simulink model "carsim_vxvy_force"  (R2021a)
settings: Solver=ode45  StartTime=0.0  StopTime=25  RelTol=1e-4
model workspace (MAT data in the model file):
  Freq = 1
values from neighbouring files (symbols this model uses):
  actuator_param = [mu_steer wn_steer csi_steer tau_steer mu_force wn_force csi_force tau_force]    [singletrack_beta_force_fialawos_ideal.m]    (also in singletrack_beta_force_fialawos_real.m; singletrack_beta_force_fialaws_ideal.m; singletrack_beta_force_fialaws_real.m; singletrack_beta_force_linear_ideal.m)
  car_param = [a b m mu Cf Cr Iz]    [singletrack_beta_force_fialawos_ideal.m]    (also in singletrack_beta_force_fialawos_real.m; singletrack_beta_force_fialaws_ideal.m; singletrack_beta_force_fialaws_real.m; singletrack_beta_force_linear_ideal.m)
  Fxr_ref = timeseries(ode_res.Fxr_ref,ode_res.t)    [singletrack_beta_force_fialawos_ideal.m]    (also in singletrack_beta_force_fialawos_real.m; singletrack_beta_force_fialaws_ideal.m; singletrack_beta_force_fialaws_real.m; singletrack_beta_force_linear_ideal.m)
  initial_state = [v0 beta0 r0 psi0 x0 y0]    [singletrack_beta_force_fialawos_ideal.m]    (also in singletrack_beta_force_fialawos_real.m; singletrack_beta_force_fialaws_ideal.m; singletrack_beta_force_fialaws_real.m; singletrack_beta_force_linear_ideal.m)
  steer_ref = timeseries(ode_res.steer_ref,ode_res.t)    [singletrack_beta_force_fialawos_ideal.m]    (also in singletrack_beta_force_fialawos_real.m; singletrack_beta_force_fialaws_ideal.m; singletrack_beta_force_fialaws_real.m; singletrack_beta_force_linear_ideal.m)
  Ts = ode_res.t(2)-ode_res.t(1)    [singletrack_beta_force_fialawos_ideal.m]    (also in singletrack_beta_force_fialawos_real.m; singletrack_beta_force_fialaws_ideal.m; singletrack_beta_force_fialaws_real.m; singletrack_beta_force_linear_ideal.m)
  tyre_model = 2    [singletrack_beta_force_fialawos_ideal.m]    (also in singletrack_beta_force_fialawos_real.m; singletrack_beta_force_fialaws_ideal.m = 1; singletrack_beta_force_fialaws_real.m = 1; singletrack_beta_force_linear_ideal.m = 0)
settings Model: Creator=bascetta  LastModifiedBy=bascetta
settings SolverCC: AlgebraicLoopSolver=TrustRegion  DecoupledContinuousIntegration=on
settings DataIOCC: SaveOutput=off  SignalLogging=off  DSMLogging=off  SaveTime=off  ReturnWorkspaceOutputs=off
settings DebuggingCC: ReadBeforeWriteMsg=DisableAll  WriteAfterWriteMsg=DisableAll  WriteAfterReadMsg=DisableAll  MultiTaskDSMMsg=none  SFMachineParentedDataDiag=warning  ArithmeticOperatorsInVariantConditions=warning
settings ModelReferenceCC: UpdateModelReferenceTargets=IfOutOfDate
settings SFSimCC: SFSimEcho=off  SimUseLocalCustomCode=off  CustomCodeUndefinedFunction=UseInterfaceOnly
settings RTWCC: RTWUseLocalCustomCode=off

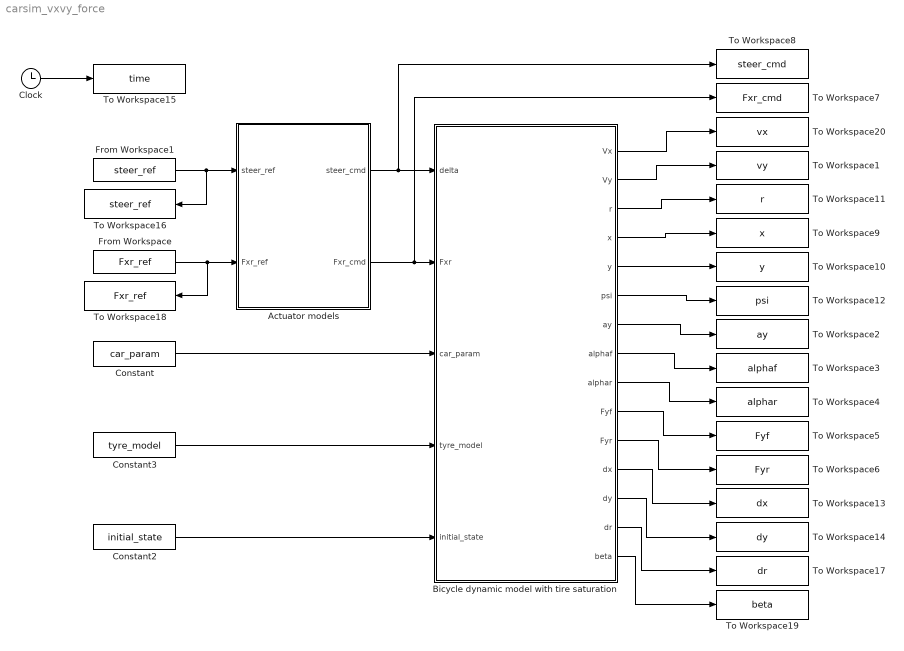
== system carsim_vxvy_force ==
  Actuator models : Subsystem  mask{mu_steer=actuator_param(1), wn_steer=actuator_param(2), csi_steer=actuator_param(3), tau_steer=actuator_param(4), steer_initial=steer_ref.Data(1), mu_force=actuator_param(5), wn_force=actuator_param(6), csi_force=actuator_param(7), tau_force=actuator_param(8), force_initial=Fxr_ref.Data(1)}
      mask prompts: mu_steer "Gain"; wn_steer "Natural frequency"; csi_steer "Damping"; tau_steer "Delay"; steer_initial "Initial value"; mu_force "Gain"; wn_force "Natural frequency"; csi_force "Damping"; tau_force "Delay"; force_initial "Initial value"
      mask DialogControl Container3 Prompt: Steer actuator parameters
      mask DialogControl Container4 Prompt: Speed actuator parameters
  Bicycle dynamic model with tire saturation : Subsystem
  Clock : Clock
  Constant : Constant  Value=car_param
  Constant2 : Constant  Value=initial_state
  Constant3 : Constant  Value=tyre_model
  From Workspace : FromWorkspace  VariableName=Fxr_ref
  From Workspace1 : FromWorkspace  VariableName=steer_ref
  To Workspace1 : ToWorkspace  VariableName=vy  SampleTime=Ts
      settings: Save2DSignal=2-D array (concatenate along first dimension)
  To Workspace10 : ToWorkspace  VariableName=y  SampleTime=Ts
      settings: Save2DSignal=2-D array (concatenate along first dimension)
  To Workspace11 : ToWorkspace  VariableName=r  SampleTime=Ts
      settings: Save2DSignal=2-D array (concatenate along first dimension)
  To Workspace12 : ToWorkspace  VariableName=psi  SampleTime=Ts
      settings: Save2DSignal=2-D array (concatenate along first dimension)
  To Workspace13 : ToWorkspace  VariableName=dx  SampleTime=Ts
      settings: Save2DSignal=2-D array (concatenate along first dimension)
  To Workspace14 : ToWorkspace  VariableName=dy  SampleTime=Ts
      settings: Save2DSignal=2-D array (concatenate along first dimension)
  To Workspace15 : ToWorkspace  VariableName=time  SampleTime=Ts
      settings: Save2DSignal=2-D array (concatenate along first dimension)
  To Workspace16 : ToWorkspace  VariableName=steer_ref  SampleTime=Ts
      settings: Save2DSignal=2-D array (concatenate along first dimension)
  To Workspace17 : ToWorkspace  VariableName=dr  SampleTime=Ts
      settings: Save2DSignal=2-D array (concatenate along first dimension)
  To Workspace18 : ToWorkspace  VariableName=Fxr_ref  SampleTime=Ts
      settings: Save2DSignal=2-D array (concatenate along first dimension)
  To Workspace19 : ToWorkspace  VariableName=beta  SampleTime=Ts
      settings: Save2DSignal=2-D array (concatenate along first dimension)
  To Workspace2 : ToWorkspace  VariableName=ay  SampleTime=Ts
      settings: Save2DSignal=2-D array (concatenate along first dimension)
  To Workspace20 : ToWorkspace  VariableName=vx  SampleTime=Ts
      settings: Save2DSignal=2-D array (concatenate along first dimension)
  To Workspace3 : ToWorkspace  VariableName=alphaf  SampleTime=Ts
      settings: Save2DSignal=2-D array (concatenate along first dimension)
  To Workspace4 : ToWorkspace  VariableName=alphar  SampleTime=Ts
      settings: Save2DSignal=2-D array (concatenate along first dimension)
  To Workspace5 : ToWorkspace  VariableName=Fyf  SampleTime=Ts
      settings: Save2DSignal=2-D array (concatenate along first dimension)
  To Workspace6 : ToWorkspace  VariableName=Fyr  SampleTime=Ts
      settings: Save2DSignal=2-D array (concatenate along first dimension)
  To Workspace7 : ToWorkspace  VariableName=Fxr_cmd  SampleTime=Ts
      settings: Save2DSignal=2-D array (concatenate along first dimension)
  To Workspace8 : ToWorkspace  VariableName=steer_cmd  SampleTime=Ts
      settings: Save2DSignal=2-D array (concatenate along first dimension)
  To Workspace9 : ToWorkspace  VariableName=x  SampleTime=Ts
      settings: Save2DSignal=2-D array (concatenate along first dimension)
  wires:
  Bicycle dynamic model with tire saturation/2(Vy) -> To Workspace1/1
  Bicycle dynamic model with tire saturation/3(r) -> To Workspace11/1
  Bicycle dynamic model with tire saturation/7(ay) -> To Workspace2/1
  Bicycle dynamic model with tire saturation/8(alphaf) -> To Workspace3/1
  Bicycle dynamic model with tire saturation/9(alphar) -> To Workspace4/1
  Bicycle dynamic model with tire saturation/10(Fyf) -> To Workspace5/1
  Bicycle dynamic model with tire saturation/11(Fyr) -> To Workspace6/1
  Constant/1 -> Bicycle dynamic model with tire saturation/3(car_param)
  Constant2/1 -> Bicycle dynamic model with tire saturation/5("initial_state ")
  Constant3/1 -> Bicycle dynamic model with tire saturation/4(tyre_model)
  Actuator models/1(steer_cmd) -> To Workspace8/1, Bicycle dynamic model with tire saturation/1(delta)
  Actuator models/2(Fxr_cmd) -> To Workspace7/1, Bicycle dynamic model with tire saturation/2(Fxr)
  From Workspace/1 -> To Workspace18/1, Actuator models/2(Fxr_ref)
  From Workspace1/1 -> To Workspace16/1, Actuator models/1(steer_ref)
  Bicycle dynamic model with tire saturation/4(x) -> To Workspace9/1
  Bicycle dynamic model with tire saturation/5(y) -> To Workspace10/1
  Bicycle dynamic model with tire saturation/6(psi) -> To Workspace12/1
  Bicycle dynamic model with tire saturation/12(dx) -> To Workspace13/1
  Bicycle dynamic model with tire saturation/13(dy) -> To Workspace14/1
  Clock/1 -> To Workspace15/1
  Bicycle dynamic model with tire saturation/14(dr) -> To Workspace17/1
  Bicycle dynamic model with tire saturation/15(beta) -> To Workspace19/1
  Bicycle dynamic model with tire saturation/1(Vx) -> To Workspace20/1

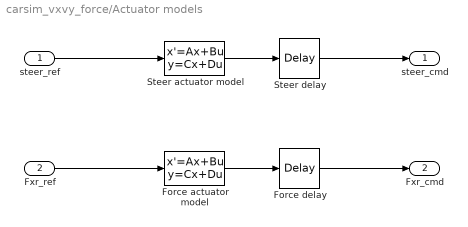
== system carsim_vxvy_force/Actuator models ==
  steer_ref : Inport
  Fxr_ref : Inport  Port=2
  Force actuator model : StateSpace  A=[0, 1; -wn_force^2, -2*csi_force*wn_force]  B=[0; mu_force*wn_force^2]  C=[1, 0]  D=0  InitialCondition=[force_initial, 0]
  Force delay : TransportDelay  DelayTime=tau_force  InitialOutput=force_initial
  Steer actuator model : StateSpace  A=[0, 1; -wn_steer^2, -2*csi_steer*wn_steer]  B=[0; mu_steer*wn_steer^2]  C=[1, 0]  D=0  InitialCondition=[steer_initial, 0]
  Steer delay : TransportDelay  DelayTime=tau_steer  InitialOutput=steer_initial
  steer_cmd : Outport
  Fxr_cmd : Outport  Port=2
  wires:
  Fxr_ref/1 -> Force actuator model/1
  Steer actuator model/1 -> Steer delay/1
  Force actuator model/1 -> Force delay/1
  steer_ref/1 -> Steer actuator model/1
  Steer delay/1 -> steer_cmd/1
  Force delay/1 -> Fxr_cmd/1

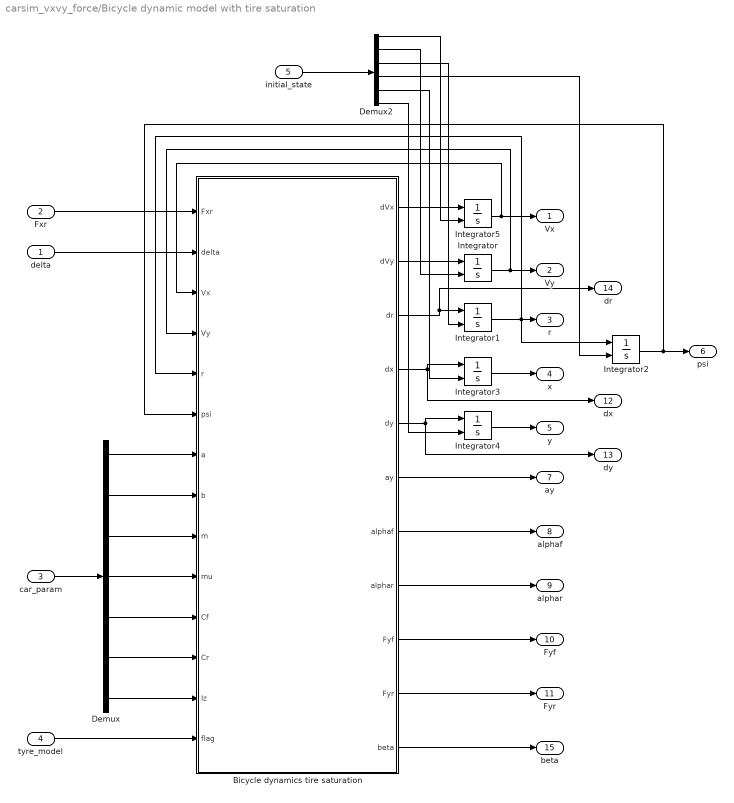
== system carsim_vxvy_force/Bicycle dynamic model with tire saturation ==
  delta : Inport
  Fxr : Inport  Port=2
  car_param : Inport  Port=3
  tyre_model : Inport  Port=4
  "initial_state " : Inport  Port=5
  Bicycle dynamics tire saturation : MATLAB Function  TreatAsAtomicUnit=on
  Demux : Demux  Outputs=7
  Demux2 : Demux  Outputs=6
  Integrator{,1..5} (6 alike) : Integrator  InitialConditionSource=external
  Vx : Outport
  Vy : Outport  Port=2
  r : Outport  Port=3
  x : Outport  Port=4
  y : Outport  Port=5
  psi : Outport  Port=6
  ay : Outport  Port=7
  alphaf : Outport  Port=8
  alphar : Outport  Port=9
  Fyf : Outport  Port=10
  Fyr : Outport  Port=11
  dx : Outport  Port=12
  dy : Outport  Port=13
  dr : Outport  Port=14
  beta : Outport  Port=15
  wires:
  Fxr/1 -> Bicycle dynamics tire saturation/1(Fxr)
  delta/1 -> Bicycle dynamics tire saturation/2(delta)
  Bicycle dynamics tire saturation/2(dVy) -> Integrator/1
  Bicycle dynamics tire saturation/3(dr) -> dr/1, Integrator1/1
  Integrator/1 -> Bicycle dynamics tire saturation/4(Vy), Vy/1
  Integrator1/1 -> Bicycle dynamics tire saturation/5(r), r/1, Integrator2/1
  Bicycle dynamics tire saturation/6(ay) -> ay/1
  Bicycle dynamics tire saturation/7(alphaf) -> alphaf/1
  Bicycle dynamics tire saturation/8(alphar) -> alphar/1
  Bicycle dynamics tire saturation/9(Fyf) -> Fyf/1
  Bicycle dynamics tire saturation/10(Fyr) -> Fyr/1
  car_param/1 -> Demux/1
  Demux/1 -> Bicycle dynamics tire saturation/7(a)
  Demux/2 -> Bicycle dynamics tire saturation/8(b)
  Demux/3 -> Bicycle dynamics tire saturation/9(m)
  Demux/4 -> Bicycle dynamics tire saturation/10(mu)
  "initial_state "/1 -> Demux2/1
  Demux2/2 -> Integrator/2
  Demux2/3 -> Integrator1/2
  tyre_model/1 -> Bicycle dynamics tire saturation/14(flag)
  Demux/5 -> Bicycle dynamics tire saturation/11(Cf)
  Demux/6 -> Bicycle dynamics tire saturation/12(Cr)
  Demux/7 -> Bicycle dynamics tire saturation/13(Iz)
  Bicycle dynamics tire saturation/4(dx) -> Integrator3/1, dx/1
  Bicycle dynamics tire saturation/5(dy) -> Integrator4/1, dy/1
  Integrator3/1 -> x/1
  Integrator4/1 -> y/1
  Demux2/4 -> Integrator2/2
  Demux2/5 -> Integrator3/2
  Demux2/6 -> Integrator4/2
  Integrator2/1 -> Bicycle dynamics tire saturation/6(psi), psi/1
  Bicycle dynamics tire saturation/11(beta) -> beta/1
  Bicycle dynamics tire saturation/1(dVx) -> Integrator5/1
  Demux2/1 -> Integrator5/2
  Integrator5/1 -> Bicycle dynamics tire saturation/3(Vx), Vx/1

== matlab function carsim_vxvy_force/Bicycle dynamic model with tire saturation/Bicycle dynamics tire saturation ==
  data: dVx output; dVy output; Fxr input; dr output; dx output; dy output; delta input; Vx input; Vy input; r input; psi input; a input; b input; m input; mu input; Cf input; Cr input; Iz input; ay output; alphaf output; alphar output; Fyf output; Fyr output; flag input; beta output
function [dVx,dVy,dr,dx,dy,ay,alphaf,alphar,Fyf,Fyr,beta]  = bicycle_dynamics(Fxr, delta, Vx, Vy, r, psi, a, b, m, mu, Cf, Cr, Iz, flag)

Fzf = m*9.81*b/(a+b);
Fzr = m*9.81*a/(a+b);

if (abs(Vx)<=0.01)
    alphaf = 0;
    alphar = 0;
else
    alphaf = atan((Vy+a*r)/Vx)-delta;
    alphar = atan((Vy-b*r)/Vx);
end

zf = tan(alphaf);
zr = tan(alphar);

zf_sl = 3*mu*Fzf/Cf;
zr_sl = 3*mu*Fzr/Cr;

switch flag
    case 0 % Linear tyre model
        Fyf = -Cf*alphaf;
        Fyr = -Cr*alphar;
    case 1 % Fiala model with saturation
        if (abs(zf)<zf_sl)
            Fyf = Cf*zf*(-1+abs(zf)/zf_sl-zf^2/(3*zf_sl^2));
        else
            Fyf = -mu*Fzf*sign(alphaf);
        end
        if (abs(zr)<zr_sl)
            Fyr = Cr*zr*(-1+abs(zr)/zr_sl-zr^2/(3*zr_sl^2));
        else
            Fyr = -mu*Fzr*sign(alphar);
        end
    case 2 % Fiala model without saturation
        Fyf = Cf*zf*(-1+abs(zf)/zf_sl-zf^2/(3*zf_sl^2));
        Fyr = Cr*zr*(-1+abs(zr)/zr_sl-zr^2/(3*zr_sl^2));
    otherwise
        Fyf = 0;
        Fyr = 0;
end

Fx  = Fxr-Fyf*sin(delta);
Fy  = Fyr+Fyf*cos(delta);
Mz  = a*Fyf*cos(delta)-b*Fyr;

dr  = Mz/Iz;
dVx = Fx/m+r*Vy;
dVy = Fy/m-r*Vx;
ay  = dVy+r*Vx;

R_psi = [cos(psi), -sin(psi); sin(psi), cos(psi)];
dx  = R_psi(1,1:2)*[Vx; Vy];
dy  = R_psi(2,1:2)*[Vx; Vy];

if (abs(Vx)<=0.01)
    beta = 0;
else
    beta = atan2(Vy,Vx);
end
